simulink model "controller"  (R2024b)
settings: Solver=ode5  StartTime=0.0  StopTime=10  FixedStep=10e-06  RelTol=1e-3
values from neighbouring files (symbols this model uses):
  K = place(Phi, Gam, z_ctrl)    [discrete_design.m]
  Nu = sol(3)    [discrete_design.m]
  Nx = sol(1:2)    [discrete_design.m]
undefined symbols (not defined in the file or in its folder): rpm2rads, u_bar_max
settings Model: Creator=Enrico  LastModifiedBy=farin
settings DataIOCC: ReturnWorkspaceOutputsName=out_black_box

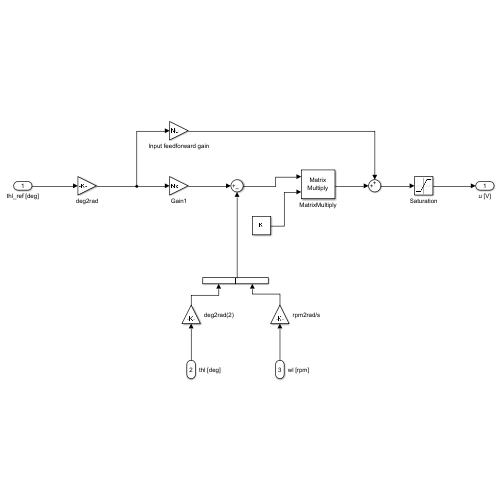
[thumbnail: Simulink's stored preview of the top-level diagram]
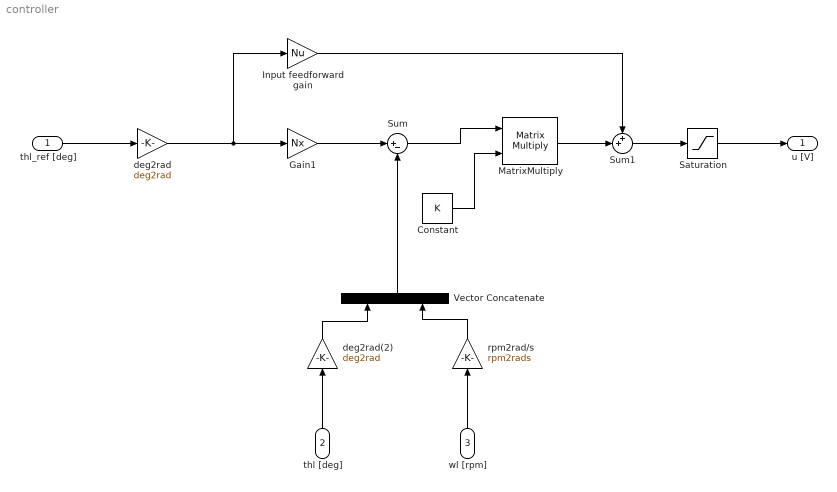
== system controller ==
  thl_ref [deg] : Inport
  thl [deg] : Inport  Port=2
  wl [rpm] : Inport  Port=3
  Constant : Constant  Value=K
  Gain1 : Gain  Gain=Nx
  Input feedforward gain : Gain  Gain=Nu
  MatrixMultiply : Product  Multiplication=Matrix(*)
  Saturation : Saturate  UpperLimit=u_bar_max  LowerLimit=-u_bar_max
  Sum : Sum  Inputs=|+-
  Sum1 : Sum  Inputs=++|
  Vector Concatenate : Concatenate
  deg2rad : Gain  Gain=deg2rad
  deg2rad(2) : Gain  Gain=deg2rad
  rpm2rad/s : Gain  Gain=rpm2rads
  u [V] : Outport
  wires:
  rpm2rad/s/1 -> Vector Concatenate/2
  deg2rad/1 -> Input feedforward gain/1, Gain1/1
  Gain1/1 -> Sum/1
  Input feedforward gain/1 -> Sum1/1
  Sum/1 -> MatrixMultiply/1
  thl [deg]/1 -> deg2rad(2)/1
  Constant/1 -> MatrixMultiply/2
  Sum1/1 -> Saturation/1
  wl [rpm]/1 -> rpm2rad/s/1
  Saturation/1 -> u [V]/1
  deg2rad(2)/1 -> Vector Concatenate/1
  MatrixMultiply/1 -> Sum1/2
  Vector Concatenate/1 -> Sum/2
  thl_ref [deg]/1 -> deg2rad/1
